simulink model "ict_serial"  (R2012b)
settings: Solver=FixedStepDiscrete  StartTime=0.0  StopTime=inf  FixedStep=Ts  RelTol=1e-3
values from neighbouring files (symbols this model uses):
  Ts = 1/(48000000 / 4095)    (= 8.53125e-05)    [obsGainsCalc.m]
undefined symbols (not defined in the file or in its folder): get, serial
libraries: dspspect3 x2, instrumentlib x2, dspsnks4 x2
settings Model: DataTypeOverride=Double  MinMaxOverflowLogging=ForceOff  Creator=admin  LastModifiedBy=admin
settings ConfigurationSet: Description=SimMechanics 2G

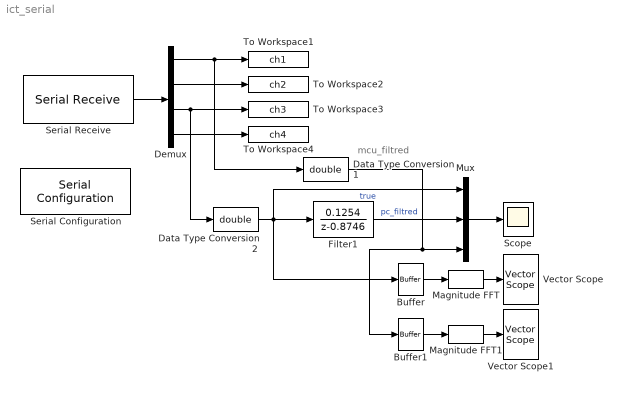
== system ict_serial ==
  note: mcu_filtred
  Buffer : Buffer  N=512  TreatMby1Signals=One channel
  Buffer1 : Buffer  N=512  TreatMby1Signals=One channel
  Data Type Conversion1 : DataTypeConversion  OutDataTypeStr=double
  Data Type Conversion2 : DataTypeConversion  OutDataTypeStr=double
  Demux : Demux
  Filter1 : DiscreteTransferFcn  Numerator=[0.1254]  Denominator=[1 -0.8746]  SampleTime=Ts  StateDataTypeStr=fixdt(1,32,16)  NumCoefDataTypeStr=fixdt(1,32,16)  DenCoefDataTypeStr=fixdt(1,32,16)  NumProductDataTypeStr=fixdt(1,32,16)  DenProductDataTypeStr=fixdt(1,32,16)  NumAccumDataTypeStr=fixdt(1,32,16)  DenAccumDataTypeStr=fixdt(1,32,16)  OutDataTypeStr=fixdt(1,32,16)  RndMeth=Round
  Magnitude FFT : dspspect3/Magnitude FFT  mag_or_magsq=Magnitude  FFTImplementation=Auto  fftLenInherit=off  fftsize=512
  Magnitude FFT1 : dspspect3/Magnitude FFT  mag_or_magsq=Magnitude  FFTImplementation=Auto  fftLenInherit=off  fftsize=512
  Mux : Mux  Inputs=3
  Scope : Scope
      settings: ShowLegends=on  YMin=-11000  YMax=11000
  Serial Configuration : instrumentlib/Serial Configuration  Priority=-200000  ComPortMenu=<Please select a port...>  ComPort=COM12  ObjConstructor=serial('COM12');  BaudRate=115200  DataBits=8  Parity=none  StopBits=1  FlowControl=none  Timeout=10  ByteOrder=LittleEndian
  Serial Receive : instrumentlib/Serial Receive  ComPortMenu=<Please select a port...>  ComPort=COM12  ObjConstructor=serial('COM12');  Header=AB  Terminator=<none>  DataSize=4  DataType=int16  EnableBlockingMode=on  ActionDataUnavailable=Output last received value  CustomValue=0  SampleTime=-1
  To Workspace1 : ToWorkspace  VariableName=ch1  SampleTime=-1
  To Workspace2 : ToWorkspace  VariableName=ch2  SampleTime=-1
  To Workspace3 : ToWorkspace  VariableName=ch3  SampleTime=-1
  To Workspace4 : ToWorkspace  VariableName=ch4  SampleTime=-1
  Vector Scope : dspsnks4/Vector Scope  ScopeProperties=on  Domain=Frequency  HorizSpan=1  DisplayProperties=off  AxisGrid=on  Memory=off  FrameNumber=on  AxisLegend=off  AxisZoom=off  OpenScopeAtSimStart=on  OpenScopeImmediately=off  FigPos=get(0,'defaultfigureposition')  AxisProperties=off  XUnits=Hertz  XRange=[0...Fs/2]  InheritXIncr=on  XIncr=1  XLabel=Time  XLimit=Auto  XMin=0  XMax=1  XStart=0  YUnits=dB  YLabel=Magnitude  LineProperties=off  XAxisParamsVer=6.9
      settings: YMin=0  YMax=100
  Vector Scope1 : dspsnks4/Vector Scope  ScopeProperties=on  Domain=Frequency  HorizSpan=1  DisplayProperties=off  AxisGrid=on  Memory=off  FrameNumber=on  AxisLegend=off  AxisZoom=off  OpenScopeAtSimStart=on  OpenScopeImmediately=off  FigPos=get(0,'defaultfigureposition')  AxisProperties=off  XUnits=Hertz  XRange=[0...Fs/2]  InheritXIncr=on  XIncr=1  XLabel=Time  XLimit=Auto  XMin=0  XMax=1  XStart=0  YUnits=dB  YLabel=Magnitude  LineProperties=off  XAxisParamsVer=6.9
      settings: YMin=0  YMax=100
  wires:
  Demux/3 -> Data Type Conversion2/1, To Workspace3/1
  Serial Receive/1 -> Demux/1
  Demux/1 -> Data Type Conversion1/1, To Workspace1/1
  Demux/2 -> To Workspace2/1
  Mux/1 -> Scope/1
  Filter1/1 -> Mux/2  "pc_filtred"
  Data Type Conversion2/1 -> Buffer/1, Filter1/1, Mux/1  "true"
  Demux/4 -> To Workspace4/1
  Data Type Conversion1/1 -> Buffer1/1, Mux/3
  Magnitude FFT/1 -> Vector Scope/1
  Buffer/1 -> Magnitude FFT/1
  Magnitude FFT1/1 -> Vector Scope1/1
  Buffer1/1 -> Magnitude FFT1/1
